simulink model "CBF_for_2Dof"  (R2024a)
settings: Solver=VariableStepAuto  StartTime=0.0  StopTime=Tf  RelTol=1e-3
undefined symbols (not defined in the file): Ts, x_init
libraries: slctrl_constraint x1
settings Model: Creator=bumyong  LastModifiedBy=bumyong

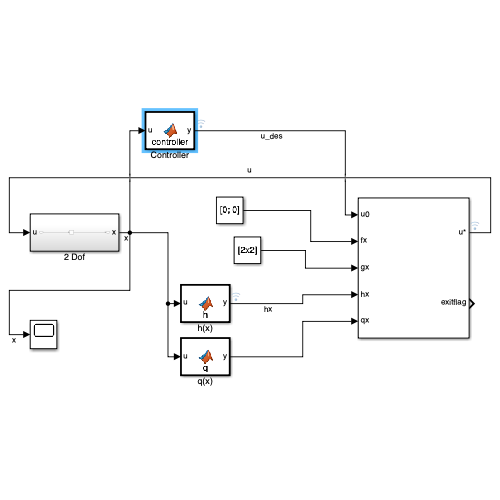
[thumbnail: Simulink's stored preview of the top-level diagram]
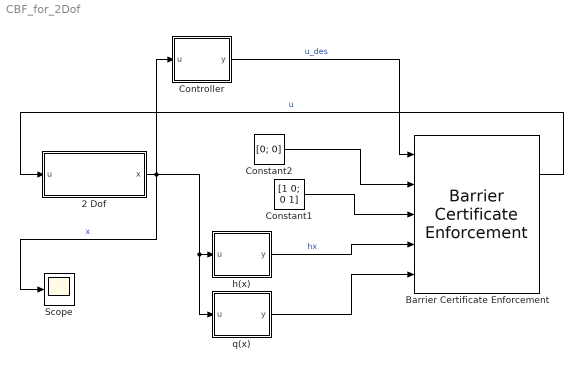
== system CBF_for_2Dof ==
  2 Dof : Subsystem
  Barrier Certificate Enforcement : slctrl_constraint/Barrier Certificate Enforcement  nx=2  nu=2  nc=1  gamma=gamma  beta=1  external_umax=off  external_umin=off  Ts=Ts  maxiter=200  tol=1e-6  output_exitflag=on
      settings: LibrarySourceBlock=slctrlblks/Constraint Control/Barrier Certificate Enforcement
  Constant1 : Constant  Value=[1 0; 0 1]
  Constant2 : Constant  Value=[0; 0]
  Controller : MATLAB Function  TreatAsAtomicUnit=on
  Scope : Scope
  h(x) : MATLAB Function  TreatAsAtomicUnit=on
  q(x) : MATLAB Function  TreatAsAtomicUnit=on
  wires:
  Barrier Certificate Enforcement/1 -> 2 Dof/1(u)  "u"
  Constant1/1 -> Barrier Certificate Enforcement/3
  2 Dof/1(x) -> Controller/1(u), Scope/1, q(x)/1(u), h(x)/1(u)  "x"
  h(x)/1(y) -> Barrier Certificate Enforcement/4  "hx"
  q(x)/1(y) -> Barrier Certificate Enforcement/5
  Constant2/1 -> Barrier Certificate Enforcement/2
  Controller/1(y) -> Barrier Certificate Enforcement/1  "u_des"

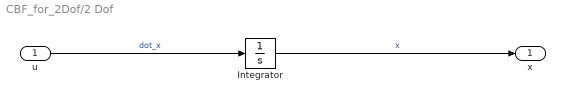
== system CBF_for_2Dof/2 Dof ==
  u : Inport
  Integrator : Integrator  InitialCondition=x_init
  x : Outport
  wires:
  u/1 -> Integrator/1  "dot_x"
  Integrator/1 -> x/1  "x"

== matlab function CBF_for_2Dof/h(x) ==
  data: u input; y output
function y = h(u)

    x = u;
    x_obs = [1; 1];
    R = 0.3;

y = norm(x - x_obs)^2 - R^2;

== matlab function CBF_for_2Dof/Controller ==
  data: u input; y output
function y = controller(u)

    x = u;
    x_tgt = [2; 2.5];
    K = 1;

y = K*(x_tgt - x);

== matlab function CBF_for_2Dof/q(x) ==
  data: u input; y output
function y = q(u)
    
x = u;

x_obs = [1; 1];



y = 2*(x-x_obs)';
